simulink subsystem "raspi_Quanser"  (R2021a)
settings: Solver=VariableStepAuto  StartTime=0.0  StopTime=10.0  RelTol=1e-3
values from neighbouring files (symbols this model uses):
  ts_raspi = 0.005    [common_data.sldd]
libraries: pendulumLib x3, SignalEditorBlockLib x2, simulink x1, raspberrypiCommlib x1
settings Model: DefaultTestHarness=raspi_Quanser_Harness1  Creator=tshintai  LastModifiedBy=tshintai

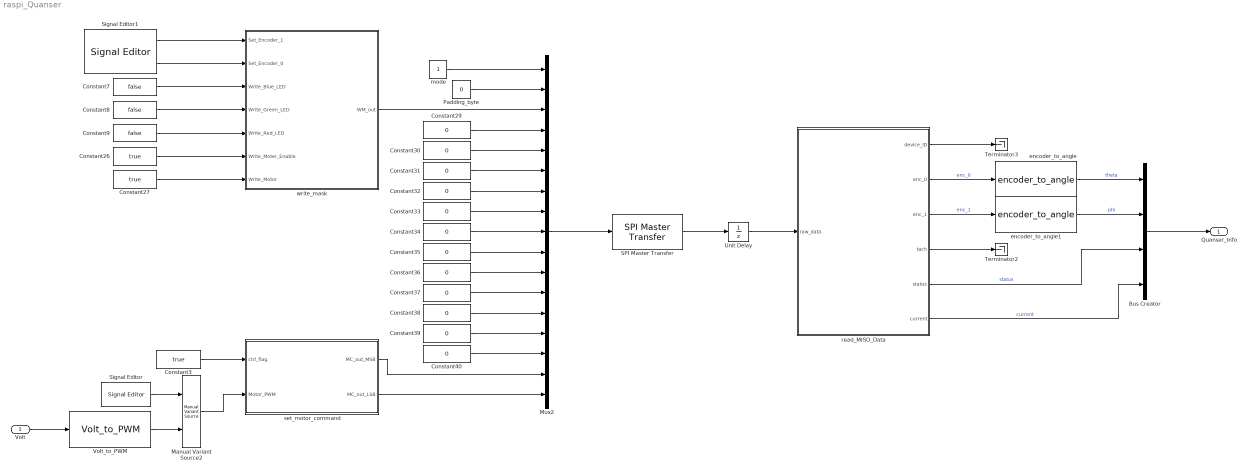
== system raspi_Quanser ==
  Volt : Inport
  Bus Creator : BusCreator  Inputs=4
  Constant26 : Constant  Value=true  SampleTime=ts_raspi
  Constant27 : Constant  Value=true  SampleTime=ts_raspi
  Constant{29..40} (12 alike) : Constant  Value=0  OutDataTypeStr=uint8  SampleTime=ts_raspi
  Constant3 : Constant  Value=true  SampleTime=ts_raspi
  Constant7 : Constant  Value=false  SampleTime=ts_raspi
  Constant8 : Constant  Value=false  SampleTime=ts_raspi
  Constant9 : Constant  Value=false  SampleTime=ts_raspi
  Manual Variant Source2 : simulink/Signal Routing/Manual Variant Source  NumChoices=2  LabelModeActiveChoice=V_2
  Mux2 : Mux  Inputs=17
  Padding_byte : Constant  Value=0  OutDataTypeStr=uint8  SampleTime=ts_raspi
  SPI Master Transfer : raspberrypiCommlib/SPI Master Transfer  BoardProperty=Pi 3 Model B+  SSPin=SPI0_CE0  SPIModule=uint32(0)  Mode=Master  BusSpeed=1000000  Pin=uint32(0)  FirstBitToTransfer=Most significant bit (MSB)  ClockMode=2  BlockFunction=Transfer  RegisterAddress=0  OutputDataType=int8  OutputDataLength=1
      settings: SourceProductBaseCode=RASPPI
  Signal Editor : SignalEditorBlockLib/Signal Editor  FileName=motor_PWM_signal.mat  ActiveScenario=No_op  ActiveSignal=Signal  IsBus=off  OutputBusObjectStr=Bus: BusObject  SampleTime=ts_raspi  Interpolate=off  ZeroCross=off  OutputAfterFinalValue=Holding final value  Unit=inherit  PreserveSignalName=on
  Signal Editor1 : SignalEditorBlockLib/Signal Editor  FileName=set_encoder_signal.mat  ActiveScenario=Scenario  ActiveSignal=Set_Encoder_1  IsBus=off  OutputBusObjectStr=Bus: BusObject  SampleTime=ts_raspi  Interpolate=off  ZeroCross=off  OutputAfterFinalValue=Holding final value  Unit=inherit  PreserveSignalName=on
  Terminator2 : Terminator
  Terminator3 : Terminator
  Unit Delay : UnitDelay  SampleTime=-1  HasFrameUpgradeWarning=on
  Volt_to_PWM : pendulumLib/Volt_to_PWM  SystemSampleTime=-1  VariantActivationTime=update diagram  Latency=0  AutoFrameSizeCalculation=off
  encoder_to_angle : pendulumLib/encoder_to_angle  SystemSampleTime=-1  VariantActivationTime=update diagram  Latency=0  AutoFrameSizeCalculation=off
  encoder_to_angle1 : pendulumLib/encoder_to_angle  SystemSampleTime=-1  VariantActivationTime=update diagram  Latency=0  AutoFrameSizeCalculation=off
  mode : Constant  OutDataTypeStr=uint8  SampleTime=ts_raspi
  read_MISO_Data : MATLAB Function  TreatAsAtomicUnit=on
  set_motor_command : MATLAB Function  TreatAsAtomicUnit=on
  write_mask : MATLAB Function  TreatAsAtomicUnit=on
  Quanser_Info : Outport
  wires:
  SPI Master Transfer/1 -> Unit Delay/1
  read_MISO_Data/2(enc_0) -> encoder_to_angle/1  "enc_0"
  read_MISO_Data/3(enc_1) -> encoder_to_angle1/1  "enc_1"
  read_MISO_Data/5(status) -> Bus Creator/3  "status"
  read_MISO_Data/6(current) -> Bus Creator/4  "current"
  read_MISO_Data/4(tach) -> Terminator2/1
  read_MISO_Data/1(device_ID) -> Terminator3/1
  encoder_to_angle/1 -> Bus Creator/1  "theta"
  encoder_to_angle1/1 -> Bus Creator/2  "phi"
  Bus Creator/1 -> Quanser_Info/1
  Signal Editor1/1 -> write_mask/1(Set_Encoder_1)
  Constant33/1 -> Mux2/8
  write_mask/1(WM_out) -> Mux2/3
  Constant34/1 -> Mux2/9
  Constant32/1 -> Mux2/7
  Constant31/1 -> Mux2/6
  Constant27/1 -> write_mask/7(Write_Motor)
  Constant7/1 -> write_mask/3(Write_Blue_LED)
  Padding_byte/1 -> Mux2/2
  Mux2/1 -> SPI Master Transfer/1
  Constant8/1 -> write_mask/4(Write_Green_LED)
  Constant3/1 -> set_motor_command/1(ctrl_flag)
  set_motor_command/2(MC_out_LSB) -> Mux2/17
  Volt/1 -> Volt_to_PWM/1
  Constant9/1 -> write_mask/5(Write_Red_LED)
  Signal Editor/1 -> Manual Variant Source2/1
  Constant29/1 -> Mux2/4
  Constant30/1 -> Mux2/5
  Manual Variant Source2/1 -> set_motor_command/2(Motor_PWM)
  Constant35/1 -> Mux2/10
  Constant40/1 -> Mux2/15
  set_motor_command/1(MC_out_MSB) -> Mux2/16
  Constant39/1 -> Mux2/14
  Constant38/1 -> Mux2/13
  Constant26/1 -> write_mask/6(Write_Moter_Enable)
  mode/1 -> Mux2/1
  Constant37/1 -> Mux2/12
  Constant36/1 -> Mux2/11
  Signal Editor1/2 -> write_mask/2(Set_Encoder_0)
  Volt_to_PWM/1 -> Manual Variant Source2/2
  Unit Delay/1 -> read_MISO_Data/1(raw_data)

== matlab function raspi_Quanser/write_mask ==
  data: Set_Encoder_1 input; WM_out output; Set_Encoder_0 input; Write_Blue_LED input; Write_Green_LED input; Write_Red_LED input; Write_Moter_Enable input; Write_Motor input
function WM_out = write_mask(Set_Encoder_1, Set_Encoder_0, ...
    Write_Blue_LED, Write_Green_LED, Write_Red_LED, ...
    Write_Moter_Enable, Write_Motor)

WM_out = uint8(0);

if Set_Encoder_1
    WM_out = bitor(WM_out, 0b01000000);
end

if Set_Encoder_0
    WM_out = bitor(WM_out, 0b00100000);
end

if Write_Blue_LED
    WM_out = bitor(WM_out, 0b00010000);
end

if Write_Green_LED
    WM_out = bitor(WM_out, 0b00001000);
end

if Write_Red_LED
    WM_out = bitor(WM_out, 0b00000100);
end

if Write_Moter_Enable
    WM_out = bitor(WM_out, 0b00000010);
end

if Write_Motor
    WM_out = bitor(WM_out, 0b00000001);
end

end

== matlab function raspi_Quanser/set_motor_command ==
  data: ctrl_flag input size=1; Motor_PWM input size=1; MC_out_MSB output uint8 size=1; MC_out_LSB output uint8 size=1
function [MC_out_MSB, MC_out_LSB] = set_motor_command(ctrl_flag, Motor_PWM)

MC = 10 * Motor_PWM;

if (MC > 999)
    MC = 999;
elseif (MC < -999)
    MC = -999;
end

MC_int = int16(MC);

MC_uint = typecast(MC_int, 'uint16');

if ctrl_flag
    MC_uint = bitor(MC_uint, uint16(0x8000));
else
    MC_uint = bitand(MC_uint, uint16(0x7FFF));
end

MC_out_MSB = uint8(bitshift(MC_uint, -8));
MC_out_LSB = uint8(bitand(MC_uint, uint16(0x00FF)));

end

== matlab function raspi_Quanser/read_MISO_Data ==
  data: raw_data input uint8 size=17; device_ID output; enc_0 output; enc_1 output; tach output; status output; current output
function [device_ID, enc_0, enc_1, ...
    tach, status, current] = read_encoder_value(raw_data)
%% Device ID
device_ID = typecast(raw_data(2:-1:1), 'uint16');

%% Encoder 0
if (raw_data(3) >= 0x80)
    last_byte = uint8(0xFF);
else
    last_byte = uint8(0x00);
end
enc_0_r = typecast([raw_data(5:-1:3); last_byte], 'int32');

enc_0 = double(enc_0_r);

%% Encoder 1
if (raw_data(6) >= 0x80)
    last_byte = uint8(0xFF);
else
    last_byte = uint8(0x00);
end
enc_1_r = typecast([raw_data(8:-1:6); last_byte], 'int32');

enc_1 = double(enc_1_r);

%% Tachometer
if (raw_data(9) >= 0x80)
    sign = 1;
else
    sign = -1;
end

r_9 = bitand(raw_data(9), 0x7F);
tach_r = typecast([raw_data(11); raw_data(10); r_9; uint8(0)], 'int32');

tach = sign * double(tach_r);

%% Status
status = raw_data(12);

%% Current Sense
current_r = typecast(raw_data(14:-1:13), 'int16');
current = double(current_r);

end
